simulink model "FAdder2"  (R2014a)
settings: Solver=ode45  StartTime=0.0  StopTime=10.0  RelTol=1e-3
settings Model: Creator=Shiyu  LastModifiedBy=Shiyu

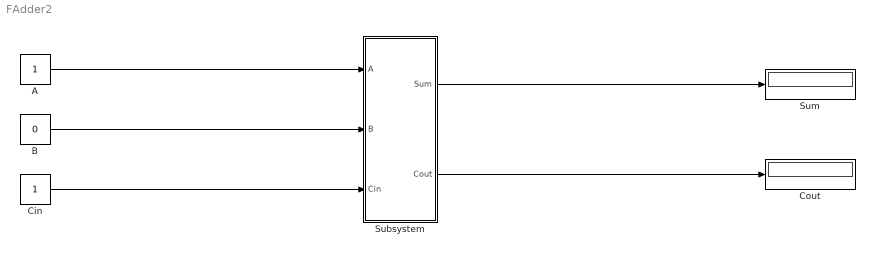
== system FAdder2 ==
  A : Constant  OutDataTypeStr=boolean
  B : Constant  Value=0  OutDataTypeStr=boolean
  Cin : Constant  OutDataTypeStr=boolean
  Cout : Display
  Subsystem : Subsystem
  "Sum " : Display
  wires:
  A/1 -> Subsystem/1(A)
  B/1 -> Subsystem/2(B)
  Cin/1 -> Subsystem/3(Cin)
  Subsystem/1(Sum) -> "Sum "/1
  Subsystem/2(Cout) -> Cout/1

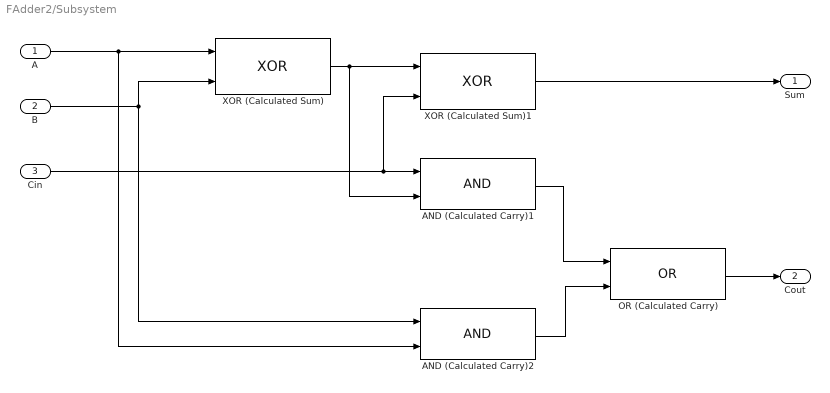
== system FAdder2/Subsystem ==
  A : Inport  OutDataTypeStr=boolean
  B : Inport  Port=2  OutDataTypeStr=boolean
  Cin : Inport  Port=3  OutDataTypeStr=boolean
  AND (Calculated Carry)1 : Logic  AllPortsSameDT=off  OutDataTypeStr=boolean
  AND (Calculated Carry)2 : Logic  AllPortsSameDT=off  OutDataTypeStr=boolean
  OR (Calculated Carry) : Logic  Operator=OR  AllPortsSameDT=off  OutDataTypeStr=boolean
  XOR (Calculated Sum) : Logic  Operator=XOR  AllPortsSameDT=off  OutDataTypeStr=boolean
  XOR (Calculated Sum)1 : Logic  Operator=XOR  AllPortsSameDT=off  OutDataTypeStr=boolean
  Sum : Outport
  Cout : Outport  Port=2
  wires:
  AND (Calculated Carry)1/1 -> OR (Calculated Carry)/1
  XOR (Calculated Sum)/1 -> AND (Calculated Carry)1/2, XOR (Calculated Sum)1/1
  OR (Calculated Carry)/1 -> Cout/1
  Cin/1 -> XOR (Calculated Sum)1/2, AND (Calculated Carry)1/1
  XOR (Calculated Sum)1/1 -> Sum/1
  A/1 -> AND (Calculated Carry)2/2, XOR (Calculated Sum)/1
  B/1 -> AND (Calculated Carry)2/1, XOR (Calculated Sum)/2
  AND (Calculated Carry)2/1 -> OR (Calculated Carry)/2
